simulink model "PostSimChalangeDavis20231208"  (R2023b)
settings: Solver=FixedStepAuto  StartTime=0.0  StopTime=inf  RelTol=1e-3  EnableMultiTasking=on
libraries: vexarmcortexlib x22, vexcommonlib x6
settings Model: Creator=carol  LastModifiedBy=User
settings SolverCC: AutoInsertRateTranBlk=on
settings DataIOCC: LimitDataPoints=on  SignalLoggingSaveFormat=ModelDataLogs  ReturnWorkspaceOutputs=off
settings OptimizationCC: ExpressionDepthLimit=2147483647  LifeSpan=Inf  MaxStackSize=64  EfficientTunableParamExpr=on
settings DebuggingCC: MergeDetectMultiDrivingBlocksExec=none  InheritedTsInSrcMsg=none  FcnCallInpInsideContextMsg=warning  StateNameClashWarn=warning  SFUnexpectedBacktrackingDiag=warning  SFNoUnconditionalDefaultTransitionDiag=warning  SFExecutionAtInitializationDiag=none  ArithmeticOperatorsInVariantConditions=warning
settings HardwareCC: ProdBitPerPointer=32  ProdBitPerSizeT=32  ProdBitPerPtrDiffT=32  ProdLargestAtomicInteger=Long  ProdLargestAtomicFloat=Double  ProdIntDivRoundTo=Undefined  ProdWordSize=32  ProdHWDeviceType=ARM Compatible->ARM Cortex
settings ModelReferenceCC: EnableRefExpFcnMdlSchedulingChecks=on  PropagateSignalLabelsOutOfModel=off
settings SFSimCC: MATLABDynamicMemAlloc=off  CustomCodeUndefinedFunction=UseInterfaceOnly
settings RTWCC: Description=Embedded Coder  SystemTargetFile=ert.tlc  HardwareBoard=ARM Cortex-based VEX Microcontroller  TemplateMakefile=ert_default_tmf  Toolchain=GNU Tools for VEX ARM Cortex
settings CodeAppCC: IgnoreCustomStorageClasses=off  CustomSymbolStrType=$N$R$M  StateflowObjectComments=on  InternalIdentifier=Classic
settings ERTTargetCC: CodeReplacementLibrary=GCC ARM Cortex-M3  MultiwordLength=2048  ConvertIfToSwitch=off  SuppressUnreachableDefaultCases=off

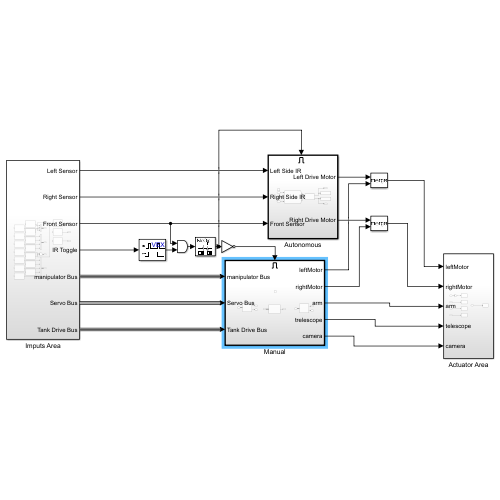
[thumbnail: Simulink's stored preview of the top-level diagram]
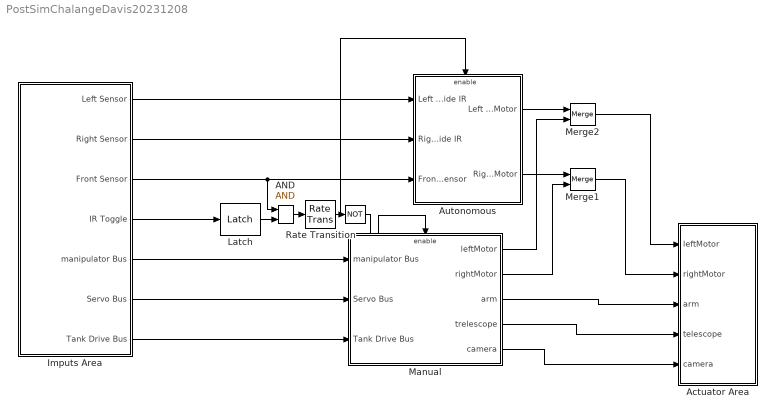
== system PostSimChalangeDavis20231208 ==
  " " : Logic  Operator=NOT  IconShape=distinctive  AllPortsSameDT=off  OutDataTypeStr=boolean
  AND : Logic  IconShape=distinctive  AllPortsSameDT=off  OutDataTypeStr=boolean
  Actuator Area : Subsystem
  Autonomous : Subsystem  TreatAsAtomicUnit=on
  Imputs Area : Subsystem
  Latch : vexcommonlib/Latch  output0=off  BlockPlatform=vexarmcortex
  Manual : Subsystem  TreatAsAtomicUnit=on
  Merge1 : Merge
  Merge2 : Merge
  Rate Transition : RateTransition
  wires:
  Manual/3(arm) -> Actuator Area/3(arm)
  Manual/5(camera) -> Actuator Area/5(camera)
  Manual/4(trelescope) -> Actuator Area/4(telescope)
  Manual/1(leftMotor) -> Merge2/2
  Manual/2(rightMotor) -> Merge1/2
  Merge1/1 -> Actuator Area/2(rightMotor)
  Merge2/1 -> Actuator Area/1(leftMotor)
  Autonomous/1(Left Drive Motor) -> Merge2/1
  Autonomous/2(Right Drive Motor) -> Merge1/1
  Imputs Area/2(Right Sensor) -> Autonomous/2(Right Side IR)
  Imputs Area/3(Front Sensor) -> Autonomous/3(Front Sensor), AND/1
  Imputs Area/1(Left Sensor) -> Autonomous/1(Left Side IR)
  Imputs Area/5(manipulator Bus) -> Manual/1(manipulator Bus)
  Imputs Area/6(Servo Bus) -> Manual/2(Servo Bus)
  Imputs Area/7(Tank Drive Bus) -> Manual/3(Tank Drive Bus)
  AND/1 -> Rate Transition/1
  Rate Transition/1 -> " "/1, Autonomous/Enable
  Imputs Area/4(IR Toggle) -> Latch/1
  Latch/1 -> AND/2
  " "/1 -> Manual/Enable

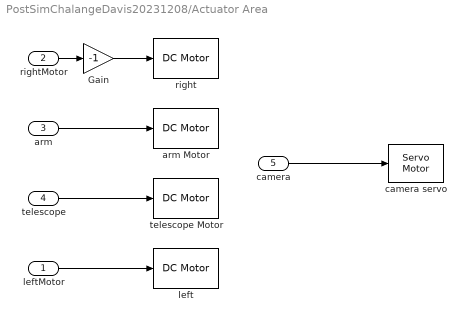
== system PostSimChalangeDavis20231208/Actuator Area ==
  leftMotor : Inport
  rightMotor : Inport  Port=2
  arm : Inport  Port=3
  telescope : Inport  Port=4
  camera : Inport  Port=5
  Gain : Gain  Gain=-1
  arm Motor : vexarmcortexlib/Actuators/DC Motor  motor=6  scaleFactor=1/13.5  SimulationOut=off
  camera servo : vexarmcortexlib/Actuators/Servo Motor  motor=7  scaleFactor=60/127  SimulationOut=off
  left : vexarmcortexlib/Actuators/DC Motor  motor=9  scaleFactor=1/13.5  SimulationOut=off
  right : vexarmcortexlib/Actuators/DC Motor  motor=2  scaleFactor=1/13.5  SimulationOut=off
  telescope Motor : vexarmcortexlib/Actuators/DC Motor  motor=5  scaleFactor=1/13.5  SimulationOut=off
  wires:
  leftMotor/1 -> left/1
  arm/1 -> arm Motor/1
  rightMotor/1 -> Gain/1
  camera/1 -> camera servo/1
  telescope/1 -> telescope Motor/1
  Gain/1 -> right/1

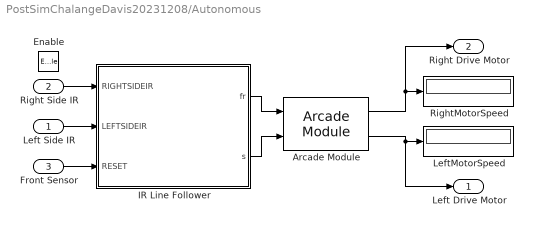
== system PostSimChalangeDavis20231208/Autonomous ==
  Left Side IR : Inport
  Right Side IR : Inport  Port=2
  Front Sensor : Inport  Port=3
  Enable : EnablePort  StatesWhenEnabling=reset
  Arcade Module : vexcommonlib/Arcade Module  BlockPlatform=vexarmcortex
  IR Line Follower : Stateflow chart  TreatAsAtomicUnit=on
  LeftMotorSpeed : Display
  RightMotorSpeed : Display
  Left Drive Motor : Outport
  Right Drive Motor : Outport  Port=2
  wires:
  Arcade Module/2 -> LeftMotorSpeed/1, Left Drive Motor/1
  Arcade Module/1 -> Right Drive Motor/1, RightMotorSpeed/1
  Front Sensor/1 -> IR Line Follower/3(RESET)
  IR Line Follower/1(fr) -> Arcade Module/1
  IR Line Follower/2(s) -> Arcade Module/2
  Right Side IR/1 -> IR Line Follower/1(RIGHTSIDEIR)
  Left Side IR/1 -> IR Line Follower/2(LEFTSIDEIR)

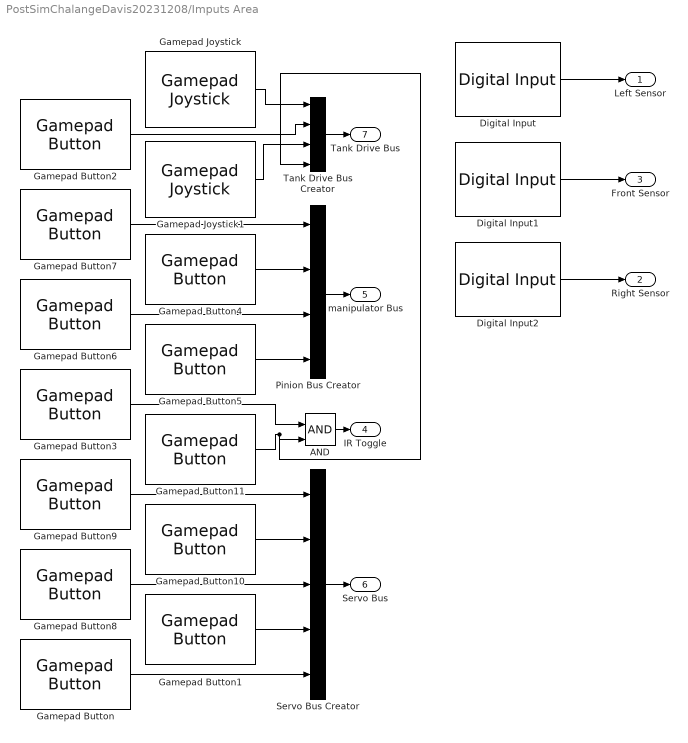
== system PostSimChalangeDavis20231208/Imputs Area ==
  AND : Logic  IconShape=distinctive  AllPortsSameDT=off  OutDataTypeStr=boolean
  Digital Input : vexarmcortexlib/Sensors/Digital Input  inChan=10  SimulationIn=on  SampleTime=0.02
  Digital Input1 : vexarmcortexlib/Sensors/Digital Input  inChan=11  SimulationIn=on  SampleTime=0.2
  Digital Input2 : vexarmcortexlib/Sensors/Digital Input  inChan=12  SimulationIn=on  SampleTime=0.02
  Gamepad Button : vexarmcortexlib/Gamepad/Gamepad Button  joystick=1  chan=7  button56=Up  button78=Left  SimulationIn=on  SampleTime=0.02
  Gamepad Button1 : vexarmcortexlib/Gamepad/Gamepad Button  joystick=1  chan=7  button56=Up  button78=Up  SimulationIn=on  SampleTime=0.02
  Gamepad Button10 : vexarmcortexlib/Gamepad/Gamepad Button  joystick=1  chan=8  button56=Up  button78=Right  SimulationIn=on  SampleTime=0.02
  Gamepad Button11 : vexarmcortexlib/Gamepad/Gamepad Button  joystick=1  chan=8  button56=Up  button78=Down  SimulationIn=on  SampleTime=0.02
  Gamepad Button2 : vexarmcortexlib/Gamepad/Gamepad Button  joystick=1  chan=7  button56=Up  button78=Right  SimulationIn=on  SampleTime=0.02
  Gamepad Button3 : vexarmcortexlib/Gamepad/Gamepad Button  joystick=1  chan=7  button56=Up  button78=Down  SimulationIn=on  SampleTime=0.02
  Gamepad Button4 : vexarmcortexlib/Gamepad/Gamepad Button  joystick=1  chan=5  button56=Down  button78=Down  SimulationIn=on  SampleTime=0.02
  Gamepad Button5 : vexarmcortexlib/Gamepad/Gamepad Button  joystick=1  chan=6  button56=Down  button78=Down  SimulationIn=on  SampleTime=0.02
  Gamepad Button6 : vexarmcortexlib/Gamepad/Gamepad Button  joystick=1  chan=6  button56=Up  button78=Down  SimulationIn=on  SampleTime=0.02
  Gamepad Button7 : vexarmcortexlib/Gamepad/Gamepad Button  joystick=1  chan=5  button56=Up  button78=Down  SimulationIn=on  SampleTime=0.02
  Gamepad Button8 : vexarmcortexlib/Gamepad/Gamepad Button  joystick=1  chan=8  button56=Up  button78=Left  SimulationIn=on  SampleTime=0.02
  Gamepad Button9 : vexarmcortexlib/Gamepad/Gamepad Button  joystick=1  chan=8  button56=Up  button78=Up  SimulationIn=on  SampleTime=0.02
  Gamepad Joystick : vexarmcortexlib/Gamepad/Gamepad Joystick  joystick=1  chan=2  SimulationIn=on  SampleTime=0.02
  Gamepad Joystick1 : vexarmcortexlib/Gamepad/Gamepad Joystick  joystick=1  chan=3  SimulationIn=on  SampleTime=0.02
  Pinion Bus Creator : BusCreator  Inputs=4
  Servo Bus Creator : BusCreator  Inputs=5
  Tank Drive Bus Creator : BusCreator  Inputs=4
  Left Sensor : Outport
  Right Sensor : Outport  Port=2
  Front Sensor : Outport  Port=3
  IR Toggle : Outport  Port=4
  manipulator Bus : Outport  Port=5
  Servo Bus : Outport  Port=6
  Tank Drive Bus : Outport  Port=7
  wires:
  Gamepad Joystick1/1 -> Tank Drive Bus Creator/3
  Gamepad Joystick/1 -> Tank Drive Bus Creator/1
  Gamepad Button9/1 -> Servo Bus Creator/1
  Gamepad Button7/1 -> Pinion Bus Creator/1
  Gamepad Button10/1 -> Servo Bus Creator/2
  Gamepad Button2/1 -> Tank Drive Bus Creator/2
  Gamepad Button6/1 -> Pinion Bus Creator/3
  Gamepad Button1/1 -> Servo Bus Creator/4
  Gamepad Button8/1 -> Servo Bus Creator/3
  Gamepad Button11/1 -> Tank Drive Bus Creator/4, AND/2
  Gamepad Button/1 -> Servo Bus Creator/5
  Gamepad Button5/1 -> Pinion Bus Creator/4
  Gamepad Button3/1 -> AND/1
  Gamepad Button4/1 -> Pinion Bus Creator/2
  Digital Input/1 -> Left Sensor/1
  Digital Input2/1 -> Right Sensor/1
  Digital Input1/1 -> Front Sensor/1
  Pinion Bus Creator/1 -> manipulator Bus/1
  Servo Bus Creator/1 -> Servo Bus/1
  Tank Drive Bus Creator/1 -> Tank Drive Bus/1
  AND/1 -> IR Toggle/1

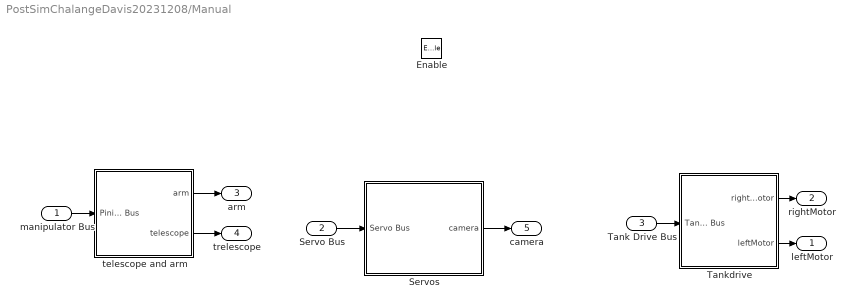
== system PostSimChalangeDavis20231208/Manual ==
  manipulator Bus : Inport
  Servo Bus : Inport  Port=2
  Tank Drive Bus : Inport  Port=3
  Enable : EnablePort
  Servos : Subsystem
  Tankdrive : Subsystem
  telescope and arm : Subsystem
  leftMotor : Outport
  rightMotor : Outport  Port=2
  arm : Outport  Port=3
  trelescope : Outport  Port=4
  camera : Outport  Port=5
  wires:
  Servos/1(camera) -> camera/1
  telescope and arm/1(arm) -> arm/1
  Servo Bus/1 -> Servos/1(Servo Bus)
  telescope and arm/2(telescope) -> trelescope/1
  manipulator Bus/1 -> telescope and arm/1(Pinion Bus)
  Tank Drive Bus/1 -> Tankdrive/1(Tank Drive Bus)
  Tankdrive/1(rightMotor) -> rightMotor/1
  Tankdrive/2(leftMotor) -> leftMotor/1

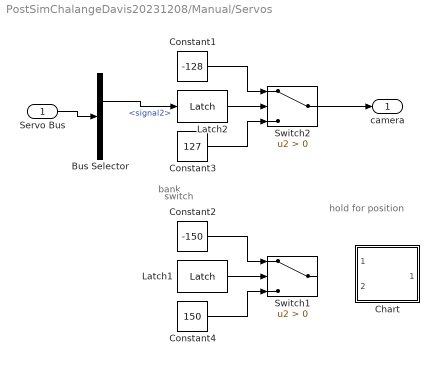
== system PostSimChalangeDavis20231208/Manual/Servos ==
  note: bank
  note: hold for position
  note: switch
  Servo Bus : Inport
  Bus Selector : BusSelector  OutputSignals=signal1,signal2,signal3,signal4,signal5
  Chart : Stateflow chart  TreatAsAtomicUnit=on
  Constant1 : Constant  Value=-128
  Constant2 : Constant  Value=-150
  Constant3 : Constant  Value=127
  Constant4 : Constant  Value=150
  Latch1 : vexcommonlib/Latch  output0=off  BlockPlatform=vexarmcortex
      settings: LibrarySourceBlock=vexarmcortexlib/Utilities/Latch
  Latch2 : vexcommonlib/Latch  output0=off  BlockPlatform=vexarmcortex
      settings: LibrarySourceBlock=vexarmcortexlib/Utilities/Latch
  Switch1 : Switch  Criteria=u2 > Threshold  SaturateOnIntegerOverflow=off  InputSameDT=off
  Switch2 : Switch  Criteria=u2 > Threshold  SaturateOnIntegerOverflow=off  InputSameDT=off
  camera : Outport
  wires:
  Servo Bus/1 -> Bus Selector/1
  Latch2/1 -> Switch2/2
  Constant1/1 -> Switch2/1
  Constant3/1 -> Switch2/3
  Constant2/1 -> Switch1/1
  Latch1/1 -> Switch1/2
  Constant4/1 -> Switch1/3
  Switch2/1 -> camera/1
  Bus Selector/2 -> Latch2/1  "<signal2>"

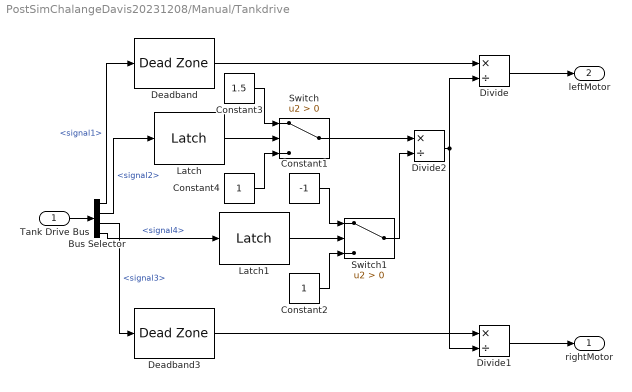
== system PostSimChalangeDavis20231208/Manual/Tankdrive ==
  Tank Drive Bus : Inport
  Bus Selector : BusSelector  OutputSignals=signal1,signal2,signal3,signal4
  Constant1 : Constant  Value=-1
  Constant2 : Constant
  Constant3 : Constant  Value=1.5
  Constant4 : Constant
  Deadband : DeadZone  LowerValue=-9  UpperValue=9
  Deadband3 : DeadZone  LowerValue=-9  UpperValue=9
  Divide : Product  Inputs=*/
  Divide1 : Product  Inputs=*/
  Divide2 : Product  Inputs=*/
  Latch : vexcommonlib/Latch  output0=off  BlockPlatform=vexarmcortex
      settings: LibrarySourceBlock=vexarmcortexlib/Utilities/Latch
  Latch1 : vexcommonlib/Latch  output0=off  BlockPlatform=vexarmcortex
      settings: LibrarySourceBlock=vexarmcortexlib/Utilities/Latch
  Switch : Switch  Criteria=u2 > Threshold  SaturateOnIntegerOverflow=off  InputSameDT=off
  Switch1 : Switch  Criteria=u2 > Threshold  SaturateOnIntegerOverflow=off  InputSameDT=off
  rightMotor : Outport
  leftMotor : Outport  Port=2
  wires:
  Constant4/1 -> Switch/3
  Constant3/1 -> Switch/1
  Divide1/1 -> rightMotor/1
  Latch/1 -> Switch/2
  Deadband3/1 -> Divide1/1
  Deadband/1 -> Divide/1
  Divide/1 -> leftMotor/1
  Tank Drive Bus/1 -> Bus Selector/1
  Bus Selector/2 -> Latch/1  "<signal2>"
  Bus Selector/1 -> Deadband/1  "<signal1>"
  Bus Selector/3 -> Deadband3/1  "<signal3>"
  Latch1/1 -> Switch1/2
  Constant2/1 -> Switch1/3
  Constant1/1 -> Switch1/1
  Bus Selector/4 -> Latch1/1  "<signal4>"
  Switch/1 -> Divide2/1
  Switch1/1 -> Divide2/2
  Divide2/1 -> Divide1/2, Divide/2

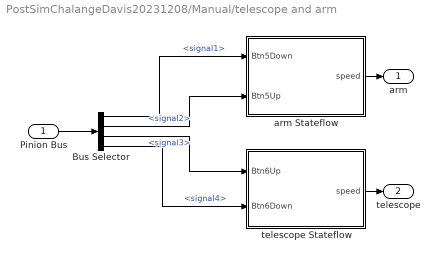
== system PostSimChalangeDavis20231208/Manual/telescope and arm ==
  Pinion Bus : Inport
  Bus Selector : BusSelector  OutputSignals=signal1,signal2,signal3,signal4
  arm Stateflow : Stateflow chart  TreatAsAtomicUnit=on
  telescope Stateflow : Stateflow chart  TreatAsAtomicUnit=on
  arm : Outport
  telescope : Outport  Port=2
  wires:
  telescope Stateflow/1(speed) -> telescope/1
  arm Stateflow/1(speed) -> arm/1
  Bus Selector/1 -> arm Stateflow/1(Btn5Down)  "<signal1>"
  Pinion Bus/1 -> Bus Selector/1
  Bus Selector/2 -> arm Stateflow/2(Btn5Up)  "<signal2>"
  Bus Selector/3 -> telescope Stateflow/1(Btn6Up)  "<signal3>"
  Bus Selector/4 -> telescope Stateflow/2(Btn6Down)  "<signal4>"

== stateflow chart PostSimChalangeDavis20231208/Manual/telescope and arm/telescope Stateflow ==
  state rackIN
    entry:
    speed=-127;
  state STOPPED
    entry:
    speed=0;
  state rackOUT
    entry:
    speed=127;
  (default) -> STOPPED
  STOPPED -> rackOUT [order 2] : [Btn6Down==0 && Btn6Up==1]
  STOPPED -> rackIN [order 1] : [Btn6Down==1 && Btn6Up==0]
  rackIN -> STOPPED [order 1] : [Btn6Down==0]
  rackOUT -> STOPPED [order 1] : [Btn6Up==0]
  rackIN -> STOPPED [order 2] : [Btn6Down==1 && Btn6Up==1]
  rackOUT -> STOPPED [order 2] : [Btn6Down==1 && Btn6Up==1]
  data: Btn6Up input; Btn6Down input; speed output

== stateflow chart PostSimChalangeDavis20231208/Manual/telescope and arm/arm Stateflow ==
  state rackIN
    entry:
    speed=-127;
  state STOPPED
    entry:
    speed=-20;
  state rackOUT
    entry:
    speed=127;
  (default) -> STOPPED
  STOPPED -> rackOUT [order 2] : [Btn5Down==0 && Btn5Up==1]
  STOPPED -> rackIN [order 1] : [Btn5Down==1 && Btn5Up==0]
  rackIN -> STOPPED [order 1] : [Btn5Down==0]
  rackOUT -> STOPPED [order 1] : [Btn5Up==0]
  rackIN -> STOPPED [order 2] : [Btn5Down==1 && Btn5Up==1]
  rackOUT -> STOPPED [order 2] : [Btn5Down==1 && Btn5Up==1]
  data: speed output; Btn5Down input; Btn5Up input

== stateflow chart PostSimChalangeDavis20231208/Autonomous/IR Line Follower ==
  state STRAIGHT
    entry:
    fr = -80;
    s = 0;
  state GO_LEFT
    entry:
    fr =0;
    s = 70;
  state GO_RIGHT
    entry:
    fr =0;
    s = -70;
  state STOP
    entry:
    fr = 0;
    s = 0;
  (default) -> STRAIGHT
  GO_LEFT -> STRAIGHT [order 3] : [LEFTSIDEIR == 0 && RIGHTSIDEIR == 0]
  GO_RIGHT -> STRAIGHT [order 3] : [RIGHTSIDEIR == 0 && LEFTSIDEIR == 0]
  STRAIGHT -> GO_RIGHT [order 2] : [RIGHTSIDEIR == 0 && LEFTSIDEIR == 1]
  STRAIGHT -> GO_LEFT [order 1] : [LEFTSIDEIR == 0 && RIGHTSIDEIR ==1]
  STOP -> STRAIGHT [order 3] : [RIGHTSIDEIR == 0 && LEFTSIDEIR == 0 && RESET == 1]
  STRAIGHT -> STOP [order 3] : [RESET == 0]
  GO_LEFT -> GO_RIGHT [order 2] : [LEFTSIDEIR == 1 && RIGHTSIDEIR == 0]
  GO_RIGHT -> GO_LEFT [order 2] : [RIGHTSIDEIR == 1 && LEFTSIDEIR == 0]
  STOP -> GO_LEFT [order 2] : [RESET == 1 && LEFTSIDEIR == 0]
  GO_LEFT -> STOP [order 1] : [RESET == 0]
  STOP -> GO_RIGHT [order 1] : [RESET == 1 && RIGHTSIDEIR == 0]
  GO_RIGHT -> STOP [order 1] : [RESET == 0]
  data: RIGHTSIDEIR input; LEFTSIDEIR input; RESET input; fr output; s output

== stateflow chart PostSimChalangeDavis20231208/Manual/Servos/Chart ==
  state neutral
    angle=3;
  state buffer
    angle=3;
  state negative40
    angle=-40;
  state positive50
    angle=50;
  (default) -> neutral
  neutral -> negative40 [order 1] : [Btn7Left==1 && Btn7Up==0]
  neutral -> positive50 [order 2] : [Btn7Up==1 && Btn7Left==0]
  buffer -> neutral : [after(.75,sec)]
  negative40 -> buffer [order 1] : [Btn7Left==1 && Btn7Up==1]
  positive50 -> buffer [order 1] : [Btn7Up==1 && Btn7Left==1]
  negative40 -> positive50 [order 2] : [Btn7Left==0 && Btn7Up==1]
  positive50 -> negative40 [order 2] : [Btn7Up==0 && Btn7Left==1]
  data: Btn7Up input; Btn7Left input; angle output
